simulink model "task1_2"  (R2020a)
settings: Solver=VariableStepAuto  StartTime=0.0  StopTime=tf  RelTol=1e-3
values from neighbouring files (symbols this model uses):
  C = transl(transl(p560.fkine(qn)))    [task1_2_script.m]
  R = 0.2    [task1_2_script.m]
libraries: roblocks x3
settings Model: Creator=root  LastModifiedBy=root

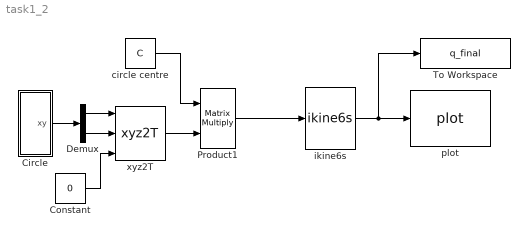
== system task1_2 ==
  Circle : Subsystem  mask{radius=R, freq=0.05}
      mask prompts: freq "Frequency (rev/s)"
  Constant : Constant  Value=0
  Demux : Demux  Outputs=2
  Product1 : Product  Multiplication=Matrix(*)  InputSameDT=on  RndMeth=Zero  SaturateOnIntegerOverflow=on  OutDataTypeStr=Inherit: Same as first input
  To Workspace : ToWorkspace  VariableName=q_final  SaveFormat=Timeseries  SampleTime=-1
  circle centre : Constant  Value=C
  ikine6s : roblocks/Arm/ikine6s  robot=p560  conf='luf'
  plot : roblocks/Arm/plot  robot=p560  fps=5  holdplot=on
  xyz2T : roblocks/Toolbox/xyz2T
  wires:
  xyz2T/1 -> Product1/2
  Demux/2 -> xyz2T/2
  Circle/1(xy) -> Demux/1
  Demux/1 -> xyz2T/1
  Constant/1 -> xyz2T/3
  Product1/1 -> ikine6s/1
  circle centre/1 -> Product1/1
  ikine6s/1 -> To Workspace/1, plot/1

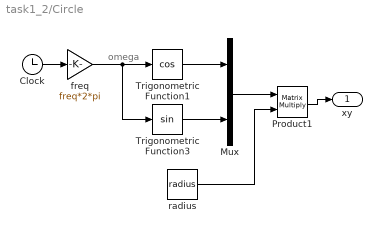
== system task1_2/Circle ==
  note: omega
  Clock : Clock
  Mux : Mux  Inputs=2
  Product1 : Product  Multiplication=Matrix(*)  RndMeth=Zero
  Trigonometric Function1 : Trigonometry  Operator=cos
  Trigonometric Function3 : Trigonometry
  freq : Gain  Gain=freq*2*pi
  radius : Constant  Value=radius
  xy : Outport
  wires:
  freq/1 -> Trigonometric Function3/1, Trigonometric Function1/1
  Product1/1 -> xy/1
  Clock/1 -> freq/1
  radius/1 -> Product1/2
  Mux/1 -> Product1/1
  Trigonometric Function1/1 -> Mux/1
  Trigonometric Function3/1 -> Mux/2
